simulink model "gm_Delay_compensation_FCS_MPC_6Phase_PMSM"  (R2022a)
settings: Solver=FixedStepDiscrete  StartTime=0.0  StopTime=10.0  RelTol=1e-3
undefined symbols (not defined in the file or in its folder): f_c, L_d, L_q, L_x, L_y, p, psi_pm, R_ph
libraries: hdlmdlgenlib x5
settings Model: Creator=Andre Merx  LastModifiedBy=Andre Merx
settings SolverCC: AlgebraicLoopSolver=TrustRegion
settings DataIOCC: LimitDataPoints=on  SaveOutput=off  SaveTime=off
settings OptimizationCC: BlockReduction=off  ConditionallyExecuteInputs=off  DefaultParameterBehavior=Inlined  LifeSpan=inf
settings DebuggingCC: AlgebraicLoopMsg=error  InheritedTsInSrcMsg=none  SingleTaskRateTransMsg=error  UnconnectedInputMsg=warning  UnconnectedOutputMsg=warning  UnconnectedLineMsg=warning  AllowSymbolicDim=off  StrictBusMsg=ErrorOnBusTreatedAsVector  SFUnexpectedBacktrackingDiag=warning  SFNoUnconditionalDefaultTransitionDiag=warning  SFExecutionAtInitializationDiag=none  SFMachineParentedDataDiag=warning  ArithmeticOperatorsInVariantConditions=warning
settings HardwareCC: ProdBitPerPointer=32  ProdBitPerSizeT=32  ProdBitPerPtrDiffT=32  ProdLargestAtomicFloat=None  ProdIntDivRoundTo=Undefined  ProdEndianess=Unspecified  ProdWordSize=32  ProdHWDeviceType=ASIC/FPGA->ASIC/FPGA  ProdEqTarget=off
settings SFSimCC: SimUseLocalCustomCode=off  CustomCodeUndefinedFunction=UseInterfaceOnly
settings RTWCC: RTWUseLocalCustomCode=off
settings CodeAppCC: StateflowObjectComments=on
settings GRTTargetCC: TargetLangStandard=C89/C90 (ANSI)
settings ConfigComp: CovScope=ReferencedModels  CovMetricSettings=dw  CovSaveCumulativeToWorkspaceVar=on  CovSaveSingleToWorkspaceVar=on  CovExternalEMLEnable=off  CovSFcnEnable=off

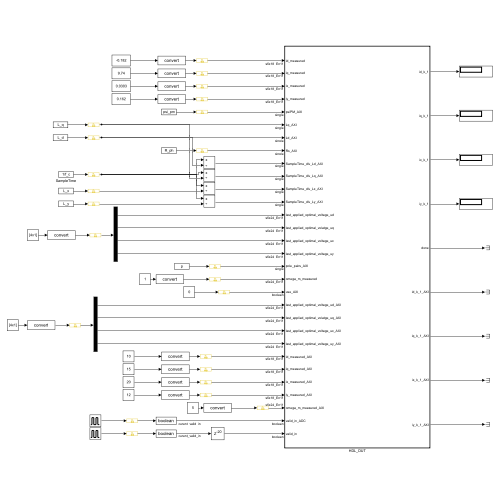
[thumbnail: Simulink's stored preview of the top-level diagram]
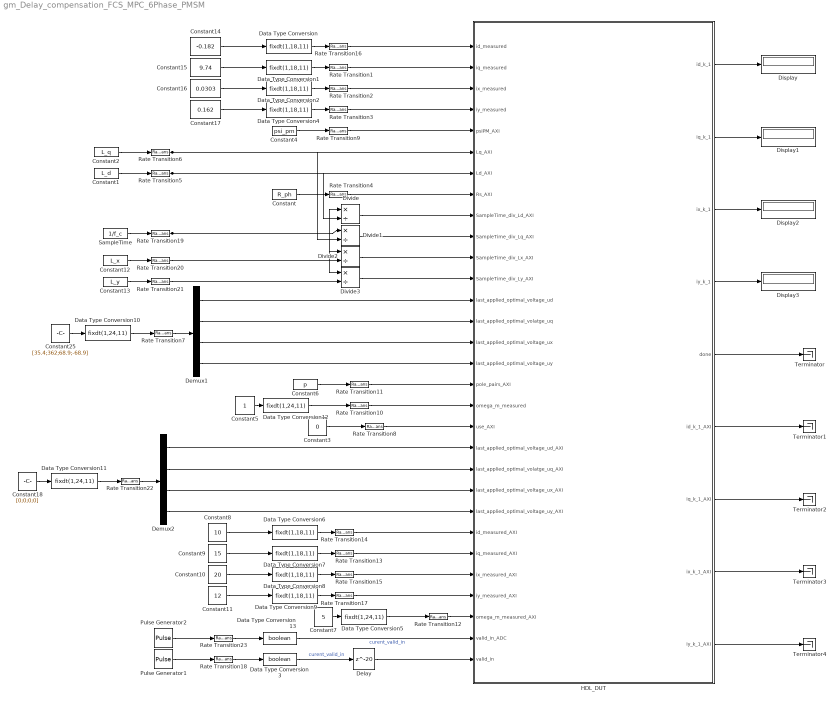
== system gm_Delay_compensation_FCS_MPC_6Phase_PMSM ==
  Constant : Constant  Value=R_ph  OutDataTypeStr=single  SampleTime=-1
  Constant1 : Constant  Value=L_d  OutDataTypeStr=single  SampleTime=-1
  Constant10 : Constant  Value=20
  Constant11 : Constant  Value=12
  Constant12 : Constant  Value=L_x  OutDataTypeStr=single  SampleTime=-1
  Constant13 : Constant  Value=L_y  OutDataTypeStr=single  SampleTime=-1
  Constant14 : Constant  Value=-0.182
  Constant15 : Constant  Value=9.74
  Constant16 : Constant  Value=0.0303
  Constant17 : Constant  Value=0.162
  Constant18 : Constant  Value=[0;0;0;0]
  Constant2 : Constant  Value=L_q  OutDataTypeStr=single  SampleTime=-1
  Constant25 : Constant  Value=[35.4;362;68.9;-68.9]
  Constant3 : Constant  Value=0  OutDataTypeStr=boolean  SampleTime=-1
  Constant4 : Constant  Value=psi_pm  OutDataTypeStr=single  SampleTime=-1
  Constant5 : Constant
  Constant6 : Constant  Value=p  OutDataTypeStr=single  SampleTime=-1
  Constant7 : Constant  Value=5
  Constant8 : Constant  Value=10
  Constant9 : Constant  Value=15
  Data Type Conversion{,1..2,4,6..9} (8 alike) : DataTypeConversion  OutDataTypeStr=fixdt(1,18,11)  SaturateOnIntegerOverflow=off  RndMeth=Floor
  Data Type Conversion{5,10..12} (4 alike) : DataTypeConversion  OutDataTypeStr=fixdt(1,24,11)  SaturateOnIntegerOverflow=off  RndMeth=Floor
  Data Type Conversion13 : DataTypeConversion  OutDataTypeStr=boolean  SaturateOnIntegerOverflow=off  RndMeth=Floor
  Data Type Conversion3 : DataTypeConversion  OutDataTypeStr=boolean  SaturateOnIntegerOverflow=off  RndMeth=Floor
  Delay : Delay  DelayLength=20
  Demux1 : Demux
  Demux2 : Demux
  Display{,1..3} (4 alike) : Display
  Divide{,1..3} (4 alike) : Product  Inputs=*/  RndMeth=Zero  SaturateOnIntegerOverflow=on
  HDL_DUT : Subsystem  TreatAsAtomicUnit=on
  Pulse Generator1 : DiscretePulseGenerator  PulseType=Time based  Period=1/f_c
  Pulse Generator2 : DiscretePulseGenerator  PulseType=Time based  Period=1/f_c
  Rate Transition{1..23} (23 alike) : RateTransition  OutPortSampleTime=Rt
  SampleTime : Constant  Value=1/f_c  OutDataTypeStr=single  SampleTime=-1
  Terminator{,1..4} (5 alike) : Terminator
  wires:
  Delay/1 -> HDL_DUT/30(valid_in)
  Data Type Conversion13/1 -> HDL_DUT/29(valid_in_ADC)  "curent_valid_in"
  Rate Transition23/1 -> Data Type Conversion13/1
  Pulse Generator2/1 -> Rate Transition23/1
  HDL_DUT/9(iy_k_1_AXI) -> Terminator4/1
  HDL_DUT/8(ix_k_1_AXI) -> Terminator3/1
  HDL_DUT/7(iq_k_1_AXI) -> Terminator2/1
  HDL_DUT/6(id_k_1_AXI) -> Terminator1/1
  Data Type Conversion11/1 -> Rate Transition22/1
  Data Type Conversion10/1 -> Rate Transition7/1
  Demux2/2 -> HDL_DUT/21(last_applied_optimal_volatge_uq_AXI)
  Demux2/4 -> HDL_DUT/23(last_applied_optimal_voltage_uy_AXI)
  Demux2/3 -> HDL_DUT/22(last_applied_optimal_voltage_ux_AXI)
  Demux2/1 -> HDL_DUT/20(last_applied_optimal_voltage_ud_AXI)
  Constant18/1 -> Data Type Conversion11/1
  Rate Transition22/1 -> Demux2/1
  Data Type Conversion7/1 -> Rate Transition13/1
  Constant9/1 -> Data Type Conversion7/1
  Rate Transition13/1 -> HDL_DUT/25(iq_measured_AXI)
  Rate Transition14/1 -> HDL_DUT/24(id_measured_AXI)
  Constant11/1 -> Data Type Conversion9/1
  Rate Transition17/1 -> HDL_DUT/27(iy_measured_AXI)
  Rate Transition15/1 -> HDL_DUT/26(ix_measured_AXI)
  Data Type Conversion9/1 -> Rate Transition17/1
  Constant8/1 -> Data Type Conversion6/1
  Data Type Conversion8/1 -> Rate Transition15/1
  Data Type Conversion6/1 -> Rate Transition14/1
  Constant10/1 -> Data Type Conversion8/1
  Rate Transition12/1 -> HDL_DUT/28(omega_m_measured_AXI)
  Data Type Conversion5/1 -> Rate Transition12/1
  Constant7/1 -> Data Type Conversion5/1
  Rate Transition8/1 -> HDL_DUT/19(use_AXI)
  Constant3/1 -> Rate Transition8/1
  HDL_DUT/5(done) -> Terminator/1
  HDL_DUT/4(iy_k_1) -> Display3/1
  HDL_DUT/3(ix_k_1) -> Display2/1
  HDL_DUT/2(iq_k_1) -> Display1/1
  HDL_DUT/1(id_k_1) -> Display/1
  Rate Transition7/1 -> Demux1/1
  Constant17/1 -> Data Type Conversion4/1
  Rate Transition16/1 -> HDL_DUT/1(id_measured)
  Constant15/1 -> Data Type Conversion1/1
  Rate Transition1/1 -> HDL_DUT/2(iq_measured)
  Data Type Conversion4/1 -> Rate Transition3/1
  Rate Transition4/1 -> HDL_DUT/8(Rs_AXI)
  Rate Transition5/1 -> HDL_DUT/7(Ld_AXI), Divide/2
  Constant6/1 -> Rate Transition11/1
  Demux1/4 -> HDL_DUT/16(last_applied_optimal_voltage_uy)
  Demux1/3 -> HDL_DUT/15(last_applied_optimal_voltage_ux)
  Constant16/1 -> Data Type Conversion2/1
  Data Type Conversion/1 -> Rate Transition16/1
  Constant4/1 -> Rate Transition9/1
  Data Type Conversion2/1 -> Rate Transition2/1
  Data Type Conversion1/1 -> Rate Transition1/1
  Constant14/1 -> Data Type Conversion/1
  Rate Transition3/1 -> HDL_DUT/4(iy_measured)
  Rate Transition2/1 -> HDL_DUT/3(ix_measured)
  Rate Transition10/1 -> HDL_DUT/18(omega_m_measured)
  Rate Transition9/1 -> HDL_DUT/5(psiPM_AXI)
  Constant5/1 -> Data Type Conversion12/1
  Data Type Conversion12/1 -> Rate Transition10/1
  Constant/1 -> Rate Transition4/1
  Rate Transition6/1 -> HDL_DUT/6(Lq_AXI), Divide1/2
  Constant1/1 -> Rate Transition5/1
  Constant2/1 -> Rate Transition6/1
  Data Type Conversion3/1 -> Delay/1  "curent_valid_in"
  Pulse Generator1/1 -> Rate Transition18/1
  Constant12/1 -> Rate Transition20/1
  Constant13/1 -> Rate Transition21/1
  Rate Transition19/1 -> Divide/1, Divide1/1, Divide2/1, Divide3/1
  Divide1/1 -> HDL_DUT/10(SampleTime_div_Lq_AXI)
  Rate Transition11/1 -> HDL_DUT/17(pole_pairs_AXI)
  Rate Transition20/1 -> Divide2/2
  Divide3/1 -> HDL_DUT/12(SampleTime_div_Ly_AXI)
  Rate Transition18/1 -> Data Type Conversion3/1
  Rate Transition21/1 -> Divide3/2
  Divide2/1 -> HDL_DUT/11(SampleTime_div_Lx_AXI)
  SampleTime/1 -> Rate Transition19/1
  Divide/1 -> HDL_DUT/9(SampleTime_div_Ld_AXI)
  Constant25/1 -> Data Type Conversion10/1
  Demux1/1 -> HDL_DUT/13(last_applied_optimal_voltage_ud)
  Demux1/2 -> HDL_DUT/14(last_applied_optimal_volatge_uq)

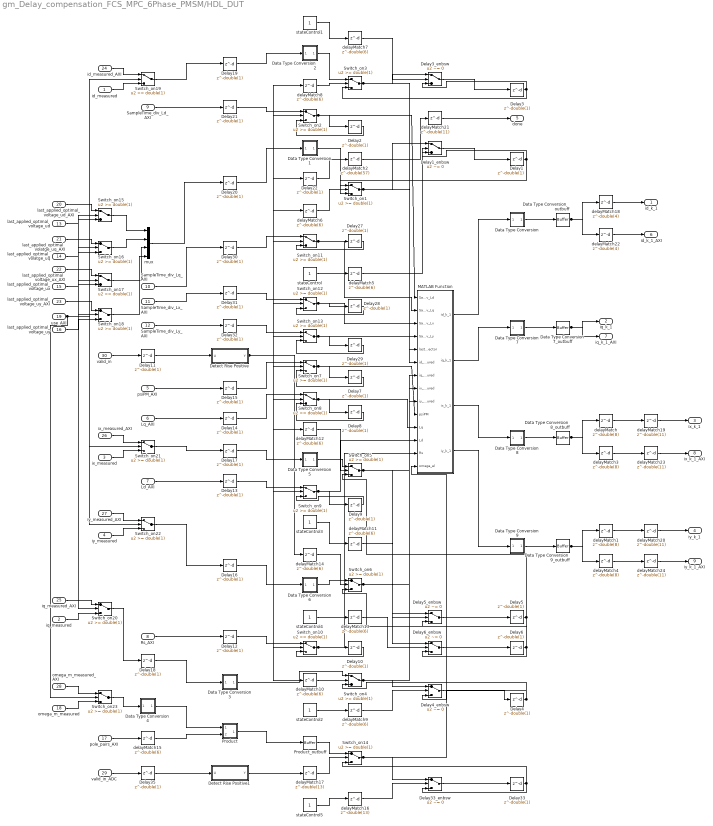
== system gm_Delay_compensation_FCS_MPC_6Phase_PMSM/HDL_DUT ==
  id_measured : Inport  OutDataTypeStr=fixdt(1, 18, 11)  PortDimensions=1  SampleTime=1e-08
  iq_measured : Inport  Port=2  OutDataTypeStr=fixdt(1, 18, 11)  PortDimensions=1  SampleTime=1e-08
  ix_measured : Inport  Port=3  OutDataTypeStr=fixdt(1, 18, 11)  PortDimensions=1  SampleTime=1e-08
  iy_measured : Inport  Port=4  OutDataTypeStr=fixdt(1, 18, 11)  PortDimensions=1  SampleTime=1e-08
  psiPM_AXI : Inport  Port=5  OutDataTypeStr=single  PortDimensions=1  SampleTime=1e-08
  Lq_AXI : Inport  Port=6  OutDataTypeStr=single  PortDimensions=1  SampleTime=1e-08
  Ld_AXI : Inport  Port=7  OutDataTypeStr=single  PortDimensions=1  SampleTime=1e-08
  Rs_AXI : Inport  Port=8  OutDataTypeStr=single  PortDimensions=1  SampleTime=1e-08
  SampleTime_div_Ld_AXI : Inport  Port=9  OutDataTypeStr=single  PortDimensions=1  SampleTime=1e-08
  SampleTime_div_Lq_AXI : Inport  Port=10  OutDataTypeStr=single  PortDimensions=1  SampleTime=1e-08
  SampleTime_div_Lx_AXI : Inport  Port=11  OutDataTypeStr=single  PortDimensions=1  SampleTime=1e-08
  SampleTime_div_Ly_AXI : Inport  Port=12  OutDataTypeStr=single  PortDimensions=1  SampleTime=1e-08
  last_applied_optimal_voltage_ud : Inport  Port=13  OutDataTypeStr=fixdt(1, 24, 11)  PortDimensions=1  SampleTime=1e-08
  last_applied_optimal_volatge_uq : Inport  Port=14  OutDataTypeStr=fixdt(1, 24, 11)  PortDimensions=1  SampleTime=1e-08
  last_applied_optimal_voltage_ux : Inport  Port=15  OutDataTypeStr=fixdt(1, 24, 11)  PortDimensions=1  SampleTime=1e-08
  last_applied_optimal_voltage_uy : Inport  Port=16  OutDataTypeStr=fixdt(1, 24, 11)  PortDimensions=1  SampleTime=1e-08
  pole_pairs_AXI : Inport  Port=17  OutDataTypeStr=single  PortDimensions=1  SampleTime=1e-08
  omega_m_measured : Inport  Port=18  OutDataTypeStr=fixdt(1, 24, 11)  PortDimensions=1  SampleTime=1e-08
  use_AXI : Inport  Port=19  OutDataTypeStr=boolean  PortDimensions=1  SampleTime=1e-08
  last_applied_optimal_voltage_ud_AXI : Inport  Port=20  OutDataTypeStr=fixdt(1, 24, 11)  PortDimensions=1  SampleTime=1e-08
  last_applied_optimal_volatge_uq_AXI : Inport  Port=21  OutDataTypeStr=fixdt(1, 24, 11)  PortDimensions=1  SampleTime=1e-08
  last_applied_optimal_voltage_ux_AXI : Inport  Port=22  OutDataTypeStr=fixdt(1, 24, 11)  PortDimensions=1  SampleTime=1e-08
  last_applied_optimal_voltage_uy_AXI : Inport  Port=23  OutDataTypeStr=fixdt(1, 24, 11)  PortDimensions=1  SampleTime=1e-08
  id_measured_AXI : Inport  Port=24  OutDataTypeStr=fixdt(1, 18, 11)  PortDimensions=1  SampleTime=1e-08
  iq_measured_AXI : Inport  Port=25  OutDataTypeStr=fixdt(1, 18, 11)  PortDimensions=1  SampleTime=1e-08
  ix_measured_AXI : Inport  Port=26  OutDataTypeStr=fixdt(1, 18, 11)  PortDimensions=1  SampleTime=1e-08
  iy_measured_AXI : Inport  Port=27  OutDataTypeStr=fixdt(1, 18, 11)  PortDimensions=1  SampleTime=1e-08
  omega_m_measured_AXI : Inport  Port=28  OutDataTypeStr=fixdt(1, 24, 11)  PortDimensions=1  SampleTime=1e-08
  valid_in_ADC : Inport  Port=29  OutDataTypeStr=boolean  PortDimensions=1  SampleTime=1e-08
  valid_in : Inport  Port=30  OutDataTypeStr=boolean  PortDimensions=1  SampleTime=1e-08
  Data Type Conversion : Subsystem
      mask Display: disp('NFP\nconv');
  Data Type Conversion1 : Subsystem
      mask Display: disp('NFP\nconv');
  Data Type Conversion2 : Subsystem
      mask Display: disp('NFP\nconv');
  Data Type Conversion3 : Subsystem
      mask Display: disp('NFP\nconv');
  Data Type Conversion4 : Subsystem
      mask Display: disp('NFP\nconv');
  Data Type Conversion5 : Subsystem
      mask Display: disp('NFP\nconv');
  Data Type Conversion6 : Subsystem
      mask Display: disp('NFP\nconv');
  Data Type Conversion7 : Subsystem
      mask Display: disp('NFP\nconv');
  Data Type Conversion7_outbuff : hdlmdlgenlib/Buffer
      settings: SourceProductBaseCode=SL
  Data Type Conversion8 : Subsystem
      mask Display: disp('NFP\nconv');
  Data Type Conversion8_outbuff : hdlmdlgenlib/Buffer
      settings: SourceProductBaseCode=SL
  Data Type Conversion9 : Subsystem
      mask Display: disp('NFP\nconv');
  Data Type Conversion9_outbuff : hdlmdlgenlib/Buffer
      settings: SourceProductBaseCode=SL
  Data Type Conversion_outbuff : hdlmdlgenlib/Buffer
      settings: SourceProductBaseCode=SL
  Delay{1..22,27..33,35} (30 alike) : Delay  DelayLength=double(1)  InitialCondition=0  SampleTime=1e-08
  Delay1_enbsw : Switch  Criteria=u2 ~= 0  Threshold=double(0)  OutDataTypeStr=single  SampleTime=1e-08  SaturateOnIntegerOverflow=off  InputSameDT=off
  Delay33_enbsw : Switch  Criteria=u2 ~= 0  Threshold=double(0)  OutDataTypeStr=single  SampleTime=1e-08  SaturateOnIntegerOverflow=off  InputSameDT=off
  Delay3_enbsw : Switch  Criteria=u2 ~= 0  Threshold=double(0)  OutDataTypeStr=single  SampleTime=1e-08  SaturateOnIntegerOverflow=off  InputSameDT=off
  Delay4_enbsw : Switch  Criteria=u2 ~= 0  Threshold=double(0)  OutDataTypeStr=single  SampleTime=1e-08  SaturateOnIntegerOverflow=off  InputSameDT=off
  Delay5_enbsw : Switch  Criteria=u2 ~= 0  Threshold=double(0)  OutDataTypeStr=single  SampleTime=1e-08  SaturateOnIntegerOverflow=off  InputSameDT=off
  Delay6_enbsw : Switch  Criteria=u2 ~= 0  Threshold=double(0)  OutDataTypeStr=single  SampleTime=1e-08  SaturateOnIntegerOverflow=off  InputSameDT=off
  Detect Rise Positive : Subsystem  mask(Detect Rise Positive){vinit=double(0), InputProcessing=Elements as channels (sample based), OutDataTypeStr=boolean}
      mask prompts: vinit "Simulink:masks:InitialCondition_MP"; InputProcessing "Simulink:masks:InputProcessing_MP"; OutDataTypeStr "Simulink:masks:OutputDataType_MP"
      mask help: Simulink:masks:DetectRisePositive_MD
      mask init:
      | InputProcessing = 'Elements as channels (sample based)';
      | OutDataTypeStr = 'boolean';
      | vinit = double(0);
      mask TypeOptions InputProcessing: Simulink:masks:ColumnsAsChannelsFrameBased | Simulink:masks:ElementsAsChannelsSampleBased
      mask TypeOptions OutDataTypeStr: Simulink:masks:uint8 | Simulink:masks:boolean
      mask Display: fprintf('U > 0\n&  NOT\nU/z > 0')
  Detect Rise Positive1 : Subsystem  mask(Detect Rise Positive){vinit=double(0), InputProcessing=Elements as channels (sample based), OutDataTypeStr=boolean}
      mask prompts: vinit "Simulink:masks:InitialCondition_MP"; InputProcessing "Simulink:masks:InputProcessing_MP"; OutDataTypeStr "Simulink:masks:OutputDataType_MP"
      mask help: Simulink:masks:DetectRisePositive_MD
      mask init:
      | InputProcessing = 'Elements as channels (sample based)';
      | OutDataTypeStr = 'boolean';
      | vinit = double(0);
      mask TypeOptions InputProcessing: Simulink:masks:ColumnsAsChannelsFrameBased | Simulink:masks:ElementsAsChannelsSampleBased
      mask TypeOptions OutDataTypeStr: Simulink:masks:uint8 | Simulink:masks:boolean
      mask Display: fprintf('U > 0\n&  NOT\nU/z > 0')
  MATLAB Function : Subsystem
  Product : Subsystem
      mask Display: disp('NFP\nmul');
  Product_outbuff : hdlmdlgenlib/Buffer
      settings: SourceProductBaseCode=SL
  Switch_on{1..14} (14 alike) : Switch  Threshold=double(1)  OutDataTypeStr=single  RndMeth=Simplest  SampleTime=1e-08  SaturateOnIntegerOverflow=off  InputSameDT=off
  Switch_on{15..18,23} (5 alike) : Switch  Threshold=double(1)  OutDataTypeStr=fixdt(1, 24, 11)  RndMeth=Simplest  SampleTime=1e-08  SaturateOnIntegerOverflow=off  InputSameDT=off
  Switch_on{19..22} (4 alike) : Switch  Threshold=double(1)  OutDataTypeStr=fixdt(1, 18, 11)  RndMeth=Simplest  SampleTime=1e-08  SaturateOnIntegerOverflow=off  InputSameDT=off
  delayMatch{,1,3..4} (4 alike) : Delay  DelayLength=double(8)  InitialCondition=0  SampleTime=1e-08
  delayMatch{5..15} (11 alike) : Delay  DelayLength=double(6)  InitialCondition=0  SampleTime=1e-08
  delayMatch16 : Delay  DelayLength=double(13)  InitialCondition=0  SampleTime=1e-08
  delayMatch17 : Delay  DelayLength=double(13)  InitialCondition=0  SampleTime=1e-08
  delayMatch18 : Delay  DelayLength=double(4)  InitialCondition=0  SampleTime=1e-08
  delayMatch{19..21,23..24} (5 alike) : Delay  DelayLength=double(11)  InitialCondition=0  SampleTime=1e-08
  delayMatch2 : Delay  DelayLength=double(57)  InitialCondition=0  SampleTime=1e-08
  delayMatch22 : Delay  DelayLength=double(4)  InitialCondition=0  SampleTime=1e-08
  mux : Mux
  stateControl{,1..5} (6 alike) : Constant  OutDataTypeStr=boolean  SampleTime=1e-08
  id_k_1 : Outport  SampleTime=1e-08
  iq_k_1 : Outport  Port=2  SampleTime=1e-08
  ix_k_1 : Outport  Port=3  SampleTime=1e-08
  iy_k_1 : Outport  Port=4  SampleTime=1e-08
  done : Outport  Port=5  SampleTime=1e-08
  id_k_1_AXI : Outport  Port=6  SampleTime=1e-08
  iq_k_1_AXI : Outport  Port=7  SampleTime=1e-08
  ix_k_1_AXI : Outport  Port=8  SampleTime=1e-08
  iy_k_1_AXI : Outport  Port=9  SampleTime=1e-08
  wires:
  id_measured/1 -> Switch_on19/3
  iq_measured/1 -> Switch_on20/3
  ix_measured/1 -> Switch_on21/3
  iy_measured/1 -> Switch_on22/3
  psiPM_AXI/1 -> Delay15/1
  Lq_AXI/1 -> Delay14/1
  Ld_AXI/1 -> Delay13/1
  Rs_AXI/1 -> Delay12/1
  SampleTime_div_Ld_AXI/1 -> Delay21/1
  SampleTime_div_Lq_AXI/1 -> Delay30/1
  SampleTime_div_Lx_AXI/1 -> Delay31/1
  SampleTime_div_Ly_AXI/1 -> Delay32/1
  last_applied_optimal_voltage_ud/1 -> Switch_on15/3
  last_applied_optimal_volatge_uq/1 -> Switch_on16/3
  last_applied_optimal_voltage_ux/1 -> Switch_on17/3
  last_applied_optimal_voltage_uy/1 -> Switch_on18/3
  delayMatch15/1 -> Product/2(In2)
  omega_m_measured/1 -> Switch_on23/3
  use_AXI/1 -> Switch_on23/2, Switch_on22/2, Switch_on21/2, Switch_on20/2, Switch_on19/2, Switch_on18/2, Switch_on17/2, Switch_on16/2, Switch_on15/2
  last_applied_optimal_voltage_ud_AXI/1 -> Switch_on15/1
  last_applied_optimal_volatge_uq_AXI/1 -> Switch_on16/1
  last_applied_optimal_voltage_ux_AXI/1 -> Switch_on17/1
  last_applied_optimal_voltage_uy_AXI/1 -> Switch_on18/1
  id_measured_AXI/1 -> Switch_on19/1
  iq_measured_AXI/1 -> Switch_on20/1
  ix_measured_AXI/1 -> Switch_on21/1
  iy_measured_AXI/1 -> Switch_on22/1
  omega_m_measured_AXI/1 -> Switch_on23/1
  valid_in_ADC/1 -> Delay35/1
  valid_in/1 -> Delay11/1
  Data Type Conversion_outbuff/1 -> delayMatch18/1, delayMatch22/1
  Data Type Conversion7_outbuff/1 -> iq_k_1_AXI/1, iq_k_1/1
  Data Type Conversion8_outbuff/1 -> delayMatch3/1, delayMatch/1
  Data Type Conversion9_outbuff/1 -> delayMatch4/1, delayMatch1/1
  Delay11/1 -> Detect Rise Positive/1(U)
  Delay12/1 -> Switch_on10/1
  Delay13/1 -> Switch_on9/1
  Delay14/1 -> Switch_on8/1
  Delay15/1 -> Switch_on7/1
  Delay16/1 -> Data Type Conversion6/1(In1)
  Delay17/1 -> Data Type Conversion5/1(In1)
  Delay18/1 -> Data Type Conversion3/1(In1)
  Delay19/1 -> Data Type Conversion2/1(In1)
  Delay20/1 -> Data Type Conversion1/1(In1)
  Delay21/1 -> Switch_on2/1
  delayMatch21/1 -> done/1
  delayMatch20/1 -> iy_k_1/1
  delayMatch19/1 -> ix_k_1/1
  delayMatch18/1 -> id_k_1/1
  Delay30/1 -> Switch_on11/1
  Delay31/1 -> Switch_on12/1
  Delay32/1 -> Switch_on13/1
  Delay35/1 -> Detect Rise Positive1/1(U)
  delayMatch6/1 -> Switch_on1/2
  delayMatch17/1 -> Switch_on14/2
  MATLAB Function/1(id_k_1) -> Data Type Conversion/1(In1)
  MATLAB Function/2(iq_k_1) -> Data Type Conversion7/1(In1)
  MATLAB Function/3(ix_k_1) -> Data Type Conversion8/1(In1)
  MATLAB Function/4(iy_k_1) -> Data Type Conversion9/1(In1)
  mux/1 -> Delay20/1
  Product_outbuff/1 -> Switch_on14/1
  Switch_on10/1 -> MATLAB Function/13(Rs), Delay10/1
  Switch_on11/1 -> MATLAB Function/2(SampleTime_div_Lq), Delay27/1
  Switch_on12/1 -> MATLAB Function/3(SampleTime_div_Lx), Delay28/1
  Switch_on13/1 -> MATLAB Function/4(SampleTime_div_Ly), Delay29/1
  Switch_on15/1 -> mux/1
  Switch_on16/1 -> mux/2
  Switch_on17/1 -> mux/3
  Switch_on18/1 -> mux/4
  Switch_on19/1 -> Delay19/1
  Switch_on2/1 -> MATLAB Function/1(SampleTime_div_Ld), Delay2/1
  Switch_on20/1 -> Delay18/1
  Switch_on21/1 -> Delay17/1
  Switch_on22/1 -> Delay16/1
  Switch_on23/1 -> Data Type Conversion4/1(In1)
  Switch_on7/1 -> MATLAB Function/10(psiPM), Delay7/1
  Switch_on8/1 -> MATLAB Function/11(Lq), Delay8/1
  Switch_on9/1 -> MATLAB Function/12(Ld), Delay9/1
  delayMatch22/1 -> id_k_1_AXI/1
  delayMatch23/1 -> ix_k_1_AXI/1
  delayMatch24/1 -> iy_k_1_AXI/1
  Delay22/1 -> delayMatch2/1
  Data Type Conversion/1(Out1) -> Data Type Conversion_outbuff/1
  Data Type Conversion1/1(Out1) -> Switch_on1/1
  Data Type Conversion2/1(Out1) -> Switch_on3/1
  Data Type Conversion3/1(Out1) -> Switch_on4/1
  Data Type Conversion4/1(Out1) -> Product/1(In1)
  Data Type Conversion5/1(Out1) -> Switch_on5/1
  Data Type Conversion6/1(Out1) -> Switch_on6/1
  Data Type Conversion7/1(Out1) -> Data Type Conversion7_outbuff/1
  Data Type Conversion8/1(Out1) -> Data Type Conversion8_outbuff/1
  Data Type Conversion9/1(Out1) -> Data Type Conversion9_outbuff/1
  Product/1(Out1) -> Product_outbuff/1
  delayMatch5/1 -> Delay1_enbsw/2
  delayMatch7/1 -> Delay3_enbsw/2
  delayMatch9/1 -> Delay4_enbsw/2
  delayMatch11/1 -> Delay5_enbsw/2
  delayMatch13/1 -> Delay6_enbsw/2
  delayMatch16/1 -> Delay33_enbsw/2
  stateControl/1 -> delayMatch5/1
  delayMatch8/1 -> Switch_on3/2
  stateControl1/1 -> delayMatch7/1
  delayMatch10/1 -> Switch_on4/2
  stateControl2/1 -> delayMatch9/1
  delayMatch12/1 -> Switch_on5/2
  stateControl3/1 -> delayMatch11/1
  delayMatch14/1 -> Switch_on6/2
  stateControl4/1 -> delayMatch13/1
  Detect Rise Positive/1(Y) -> delayMatch14/1, delayMatch12/1, delayMatch10/1, delayMatch8/1, delayMatch6/1, Delay22/1, Switch_on2/2, Switch_on11/2, Switch_on12/2, Switch_on13/2, Switch_on7/2, Switch_on8/2, Switch_on9/2, Switch_on10/2
  pole_pairs_AXI/1 -> delayMatch15/1
  stateControl5/1 -> delayMatch16/1
  Detect Rise Positive1/1(Y) -> delayMatch17/1
  delayMatch/1 -> delayMatch19/1
  delayMatch1/1 -> delayMatch20/1
  delayMatch2/1 -> delayMatch21/1
  delayMatch3/1 -> delayMatch23/1
  delayMatch4/1 -> delayMatch24/1
  Switch_on1/1 -> MATLAB Function/5(last_applied_optimal_voltage_vector), Delay1_enbsw/1
  Switch_on3/1 -> MATLAB Function/6(id_measured), Delay3_enbsw/1
  Switch_on4/1 -> MATLAB Function/7(iq_measured), Delay4_enbsw/1
  Switch_on5/1 -> MATLAB Function/8(ix_measured), Delay5_enbsw/1
  Switch_on6/1 -> MATLAB Function/9(iy_measured), Delay6_enbsw/1
  Switch_on14/1 -> MATLAB Function/14(omega_el), Delay33_enbsw/1
  Delay2/1 -> Switch_on2/3
  Delay27/1 -> Switch_on11/3
  Delay28/1 -> Switch_on12/3
  Delay29/1 -> Switch_on13/3
  Delay1_enbsw/1 -> Delay1/1
  Delay1/1 -> Switch_on1/3, Delay1_enbsw/3
  Delay3_enbsw/1 -> Delay3/1
  Delay3/1 -> Switch_on3/3, Delay3_enbsw/3
  Delay4_enbsw/1 -> Delay4/1
  Delay4/1 -> Switch_on4/3, Delay4_enbsw/3
  Delay5_enbsw/1 -> Delay5/1
  Delay5/1 -> Switch_on5/3, Delay5_enbsw/3
  Delay6_enbsw/1 -> Delay6/1
  Delay6/1 -> Switch_on6/3, Delay6_enbsw/3
  Delay7/1 -> Switch_on7/3
  Delay8/1 -> Switch_on8/3
  Delay9/1 -> Switch_on9/3
  Delay10/1 -> Switch_on10/3
  Delay33_enbsw/1 -> Delay33/1
  Delay33/1 -> Switch_on14/3, Delay33_enbsw/3

== system gm_Delay_compensation_FCS_MPC_6Phase_PMSM/HDL_DUT/Data Type Conversion ==
  In1 : Inport
  Data Type Conversion : DataTypeConversion  OutDataTypeStr=fixdt(1, 18, 11)  SampleTime=1e-08  SaturateOnIntegerOverflow=off  RndMeth=Floor
  Data Type Conversion_pd1 : Delay  DelayLength=6
  Out1 : Outport
  wires:
  In1/1 -> Data Type Conversion/1
  Data Type Conversion/1 -> Data Type Conversion_pd1/1
  Data Type Conversion_pd1/1 -> Out1/1

== system gm_Delay_compensation_FCS_MPC_6Phase_PMSM/HDL_DUT/Data Type Conversion1 ==
  In1 : Inport
  Data Type Conversion1 : DataTypeConversion  OutDataTypeStr=single  RndMeth=Nearest  SampleTime=1e-08  SaturateOnIntegerOverflow=off
  Data Type Conversion1_pd1 : Delay  DelayLength=6
  Out1 : Outport
  wires:
  In1/1 -> Data Type Conversion1/1
  Data Type Conversion1/1 -> Data Type Conversion1_pd1/1
  Data Type Conversion1_pd1/1 -> Out1/1

== system gm_Delay_compensation_FCS_MPC_6Phase_PMSM/HDL_DUT/Data Type Conversion2 ==
  In1 : Inport
  Data Type Conversion2 : DataTypeConversion  OutDataTypeStr=single  RndMeth=Nearest  SampleTime=1e-08  SaturateOnIntegerOverflow=off
  Data Type Conversion2_pd1 : Delay  DelayLength=6
  Out1 : Outport
  wires:
  In1/1 -> Data Type Conversion2/1
  Data Type Conversion2/1 -> Data Type Conversion2_pd1/1
  Data Type Conversion2_pd1/1 -> Out1/1

== system gm_Delay_compensation_FCS_MPC_6Phase_PMSM/HDL_DUT/Data Type Conversion3 ==
  In1 : Inport
  Data Type Conversion3 : DataTypeConversion  OutDataTypeStr=single  RndMeth=Nearest  SampleTime=1e-08  SaturateOnIntegerOverflow=off
  Data Type Conversion3_pd1 : Delay  DelayLength=6
  Out1 : Outport
  wires:
  In1/1 -> Data Type Conversion3/1
  Data Type Conversion3/1 -> Data Type Conversion3_pd1/1
  Data Type Conversion3_pd1/1 -> Out1/1

== system gm_Delay_compensation_FCS_MPC_6Phase_PMSM/HDL_DUT/Data Type Conversion4 ==
  In1 : Inport
  Data Type Conversion4 : DataTypeConversion  OutDataTypeStr=single  RndMeth=Nearest  SampleTime=1e-08  SaturateOnIntegerOverflow=off
  Data Type Conversion4_pd1 : Delay  DelayLength=6
  Out1 : Outport
  wires:
  In1/1 -> Data Type Conversion4/1
  Data Type Conversion4/1 -> Data Type Conversion4_pd1/1
  Data Type Conversion4_pd1/1 -> Out1/1

== system gm_Delay_compensation_FCS_MPC_6Phase_PMSM/HDL_DUT/Data Type Conversion5 ==
  In1 : Inport
  Data Type Conversion5 : DataTypeConversion  OutDataTypeStr=single  RndMeth=Nearest  SampleTime=1e-08  SaturateOnIntegerOverflow=off
  Data Type Conversion5_pd1 : Delay  DelayLength=6
  Out1 : Outport
  wires:
  In1/1 -> Data Type Conversion5/1
  Data Type Conversion5/1 -> Data Type Conversion5_pd1/1
  Data Type Conversion5_pd1/1 -> Out1/1

== system gm_Delay_compensation_FCS_MPC_6Phase_PMSM/HDL_DUT/Data Type Conversion6 ==
  In1 : Inport
  Data Type Conversion6 : DataTypeConversion  OutDataTypeStr=single  RndMeth=Nearest  SampleTime=1e-08  SaturateOnIntegerOverflow=off
  Data Type Conversion6_pd1 : Delay  DelayLength=6
  Out1 : Outport
  wires:
  In1/1 -> Data Type Conversion6/1
  Data Type Conversion6/1 -> Data Type Conversion6_pd1/1
  Data Type Conversion6_pd1/1 -> Out1/1

== system gm_Delay_compensation_FCS_MPC_6Phase_PMSM/HDL_DUT/Data Type Conversion7 ==
  In1 : Inport
  Data Type Conversion7 : DataTypeConversion  OutDataTypeStr=fixdt(1, 18, 11)  SampleTime=1e-08  SaturateOnIntegerOverflow=off  RndMeth=Floor
  Data Type Conversion7_pd1 : Delay  DelayLength=6
  Out1 : Outport
  wires:
  In1/1 -> Data Type Conversion7/1
  Data Type Conversion7/1 -> Data Type Conversion7_pd1/1
  Data Type Conversion7_pd1/1 -> Out1/1

== system gm_Delay_compensation_FCS_MPC_6Phase_PMSM/HDL_DUT/Data Type Conversion8 ==
  In1 : Inport
  Data Type Conversion8 : DataTypeConversion  OutDataTypeStr=fixdt(1, 18, 11)  SampleTime=1e-08  SaturateOnIntegerOverflow=off  RndMeth=Floor
  Data Type Conversion8_pd1 : Delay  DelayLength=6
  Out1 : Outport
  wires:
  In1/1 -> Data Type Conversion8/1
  Data Type Conversion8/1 -> Data Type Conversion8_pd1/1
  Data Type Conversion8_pd1/1 -> Out1/1

== system gm_Delay_compensation_FCS_MPC_6Phase_PMSM/HDL_DUT/Data Type Conversion9 ==
  In1 : Inport
  Data Type Conversion9 : DataTypeConversion  OutDataTypeStr=fixdt(1, 18, 11)  SampleTime=1e-08  SaturateOnIntegerOverflow=off  RndMeth=Floor
  Data Type Conversion9_pd1 : Delay  DelayLength=6
  Out1 : Outport
  wires:
  In1/1 -> Data Type Conversion9/1
  Data Type Conversion9/1 -> Data Type Conversion9_pd1/1
  Data Type Conversion9_pd1/1 -> Out1/1

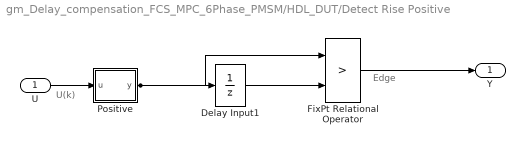
== system gm_Delay_compensation_FCS_MPC_6Phase_PMSM/HDL_DUT/Detect Rise Positive ==
  note: Edge
  note: U(k)
  U : Inport  OutDataTypeStr=boolean  SampleTime=1e-08
  Delay Input1 : UnitDelay  Description=Store in Global RAM  DisableCoverage=on  InitialCondition=vinit  SampleTime=-1  HasFrameUpgradeWarning=on
  FixPt Relational Operator : RelationalOperator  Operator=>  OutDataTypeStr=boolean  ZeroCross=off  InputSameDT=off
  Positive : Subsystem  mask(Compare To Zero){relop=>, OutDataTypeStr=boolean, ZeroCross=off}
      mask prompts: relop "Simulink:masks:Operator_MP"; OutDataTypeStr "Simulink:masks:OutputDataType_MP"; ZeroCross "Simulink:masks:EnableZerocrossingDetection_MP"
      mask help: Simulink:masks:CompareToZero_MD
      mask init:
      | OutDataTypeStr = 'boolean';
      | ZeroCross = 'off';
      | blkName = 'Delay_compensation_FCS_MPC_6Phase_PMSM/HDL_DUT/Detect Rise\nPositive/Positive';
      | relop = '>';
      | setValue = 'boolean';
      mask TypeOptions relop: == | ~= | < | <= | >= | >
      mask TypeOptions OutDataTypeStr: Simulink:masks:uint8 | Simulink:masks:boolean
      mask Callback ZeroCross: sl('zeroCrossEnable', gcbh);
      mask Display: disp([relop,' 0'])
  Y : Outport  SampleTime=1e-08
  wires:
  Delay Input1/1 -> FixPt Relational Operator/2
  FixPt Relational Operator/1 -> Y/1
  Positive/1(y) -> FixPt Relational Operator/1, Delay Input1/1
  U/1 -> Positive/1(u)

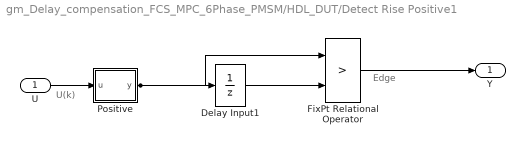
== system gm_Delay_compensation_FCS_MPC_6Phase_PMSM/HDL_DUT/Detect Rise Positive1 ==
  note: Edge
  note: U(k)
  U : Inport  OutDataTypeStr=boolean  SampleTime=1e-08
  Delay Input1 : UnitDelay  Description=Store in Global RAM  DisableCoverage=on  InitialCondition=vinit  SampleTime=-1  HasFrameUpgradeWarning=on
  FixPt Relational Operator : RelationalOperator  Operator=>  OutDataTypeStr=boolean  ZeroCross=off  InputSameDT=off
  Positive : Subsystem  mask(Compare To Zero){relop=>, OutDataTypeStr=boolean, ZeroCross=off}
      mask prompts: relop "Simulink:masks:Operator_MP"; OutDataTypeStr "Simulink:masks:OutputDataType_MP"; ZeroCross "Simulink:masks:EnableZerocrossingDetection_MP"
      mask help: Simulink:masks:CompareToZero_MD
      mask init:
      | OutDataTypeStr = 'boolean';
      | ZeroCross = 'off';
      | blkName = 'Delay_compensation_FCS_MPC_6Phase_PMSM/HDL_DUT/Detect Rise\nPositive1/Positive';
      | relop = '>';
      | setValue = 'boolean';
      mask TypeOptions relop: == | ~= | < | <= | >= | >
      mask TypeOptions OutDataTypeStr: Simulink:masks:uint8 | Simulink:masks:boolean
      mask Callback ZeroCross: sl('zeroCrossEnable', gcbh);
      mask Display: disp([relop,' 0'])
  Y : Outport  SampleTime=1e-08
  wires:
  Delay Input1/1 -> FixPt Relational Operator/2
  FixPt Relational Operator/1 -> Y/1
  Positive/1(y) -> FixPt Relational Operator/1, Delay Input1/1
  U/1 -> Positive/1(u)

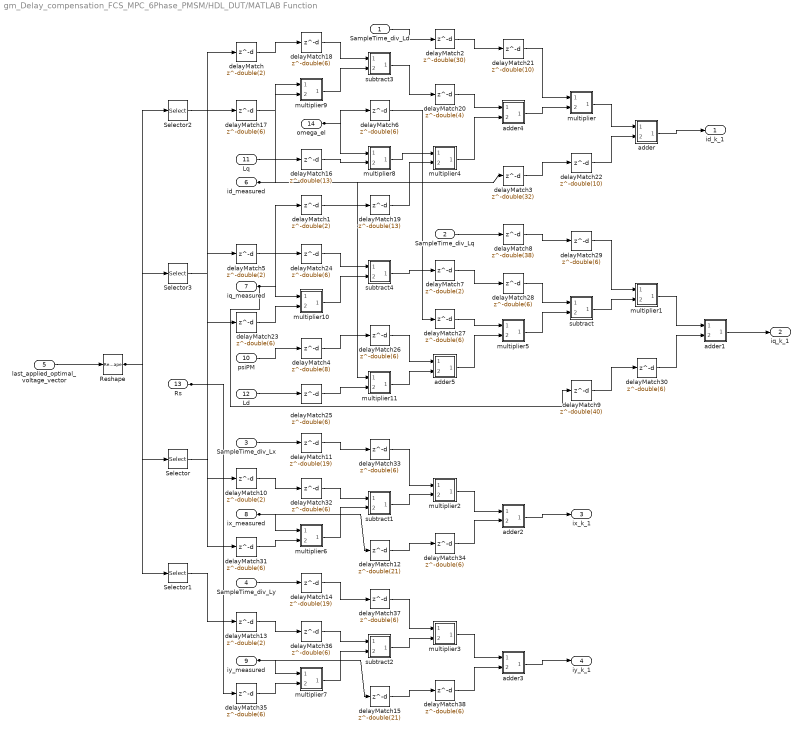
== system gm_Delay_compensation_FCS_MPC_6Phase_PMSM/HDL_DUT/MATLAB Function ==
  SampleTime_div_Ld : Inport  OutDataTypeStr=single  PortDimensions=1  SampleTime=1e-08
  SampleTime_div_Lq : Inport  Port=2  OutDataTypeStr=single  PortDimensions=1  SampleTime=1e-08
  SampleTime_div_Lx : Inport  Port=3  OutDataTypeStr=single  PortDimensions=1  SampleTime=1e-08
  SampleTime_div_Ly : Inport  Port=4  OutDataTypeStr=single  PortDimensions=1  SampleTime=1e-08
  last_applied_optimal_voltage_vector : Inport  Port=5  OutDataTypeStr=single  PortDimensions=[4]  SampleTime=1e-08
  id_measured : Inport  Port=6  OutDataTypeStr=single  PortDimensions=1  SampleTime=1e-08
  iq_measured : Inport  Port=7  OutDataTypeStr=single  PortDimensions=1  SampleTime=1e-08
  ix_measured : Inport  Port=8  OutDataTypeStr=single  PortDimensions=1  SampleTime=1e-08
  iy_measured : Inport  Port=9  OutDataTypeStr=single  PortDimensions=1  SampleTime=1e-08
  psiPM : Inport  Port=10  OutDataTypeStr=single  PortDimensions=1  SampleTime=1e-08
  Lq : Inport  Port=11  OutDataTypeStr=single  PortDimensions=1  SampleTime=1e-08
  Ld : Inport  Port=12  OutDataTypeStr=single  PortDimensions=1  SampleTime=1e-08
  Rs : Inport  Port=13  OutDataTypeStr=single  PortDimensions=1  SampleTime=1e-08
  omega_el : Inport  Port=14  OutDataTypeStr=single  PortDimensions=1  SampleTime=1e-08
  Reshape : Reshape  OutputDimensionality=Column vector (2-D)
  Selector : Selector  SampleTime=1e-08  IndexOptions=Index vector (dialog)  Indices=double(3)  OutputSizes=double(0)
  Selector1 : Selector  SampleTime=1e-08  IndexOptions=Index vector (dialog)  Indices=double(4)  OutputSizes=double(0)
  Selector2 : Selector  SampleTime=1e-08  IndexOptions=Index vector (dialog)  Indices=double(1)  OutputSizes=double(0)
  Selector3 : Selector  SampleTime=1e-08  IndexOptions=Index vector (dialog)  Indices=double(2)  OutputSizes=double(0)
  adder : Subsystem
      mask Display: disp('NFP\nadd');
  adder1 : Subsystem
      mask Display: disp('NFP\nadd');
  adder2 : Subsystem
      mask Display: disp('NFP\nadd');
  adder3 : Subsystem
      mask Display: disp('NFP\nadd');
  adder4 : Subsystem
      mask Display: disp('NFP\nadd');
  adder5 : Subsystem
      mask Display: disp('NFP\nadd');
  delayMatch{,1,5,7,10,13} (6 alike) : Delay  DelayLength=double(2)  InitialCondition=0  SampleTime=1e-08
  delayMatch11 : Delay  DelayLength=double(19)  InitialCondition=0  SampleTime=1e-08
  delayMatch12 : Delay  DelayLength=double(21)  InitialCondition=0  SampleTime=1e-08
  delayMatch14 : Delay  DelayLength=double(19)  InitialCondition=0  SampleTime=1e-08
  delayMatch15 : Delay  DelayLength=double(21)  InitialCondition=0  SampleTime=1e-08
  delayMatch16 : Delay  DelayLength=double(13)  InitialCondition=0  SampleTime=1e-08
  delayMatch{6,17..18,23..38} (19 alike) : Delay  DelayLength=double(6)  InitialCondition=0  SampleTime=1e-08
  delayMatch19 : Delay  DelayLength=double(13)  InitialCondition=0  SampleTime=1e-08
  delayMatch2 : Delay  DelayLength=double(30)  InitialCondition=0  SampleTime=1e-08
  delayMatch20 : Delay  DelayLength=double(4)  InitialCondition=0  SampleTime=1e-08
  delayMatch21 : Delay  DelayLength=double(10)  InitialCondition=0  SampleTime=1e-08
  delayMatch22 : Delay  DelayLength=double(10)  InitialCondition=0  SampleTime=1e-08
  delayMatch3 : Delay  DelayLength=double(32)  InitialCondition=0  SampleTime=1e-08
  delayMatch4 : Delay  DelayLength=double(8)  InitialCondition=0  SampleTime=1e-08
  delayMatch8 : Delay  DelayLength=double(38)  InitialCondition=0  SampleTime=1e-08
  delayMatch9 : Delay  DelayLength=double(40)  InitialCondition=0  SampleTime=1e-08
  multiplier : Subsystem
      mask Display: disp('NFP\nmul');
  multiplier1 : Subsystem
      mask Display: disp('NFP\nmul');
  multiplier10 : Subsystem
      mask Display: disp('NFP\nmul');
  multiplier11 : Subsystem
      mask Display: disp('NFP\nmul');
  multiplier2 : Subsystem
      mask Display: disp('NFP\nmul');
  multiplier3 : Subsystem
      mask Display: disp('NFP\nmul');
  multiplier4 : Subsystem
      mask Display: disp('NFP\nmul');
  multiplier5 : Subsystem
      mask Display: disp('NFP\nmul');
  multiplier6 : Subsystem
      mask Display: disp('NFP\nmul');
  multiplier7 : Subsystem
      mask Display: disp('NFP\nmul');
  multiplier8 : Subsystem
      mask Display: disp('NFP\nmul');
  multiplier9 : Subsystem
      mask Display: disp('NFP\nmul');
  subtract : Subsystem
      mask Display: disp('NFP\nadd');
  subtract1 : Subsystem
      mask Display: disp('NFP\nadd');
  subtract2 : Subsystem
      mask Display: disp('NFP\nadd');
  subtract3 : Subsystem
      mask Display: disp('NFP\nadd');
  subtract4 : Subsystem
      mask Display: disp('NFP\nadd');
  id_k_1 : Outport  SampleTime=1e-08  VectorParamsAs1DForOutWhenUnconnected=off
  iq_k_1 : Outport  Port=2  SampleTime=1e-08
  ix_k_1 : Outport  Port=3  SampleTime=1e-08
  iy_k_1 : Outport  Port=4  SampleTime=1e-08
  wires:
  delayMatch21/1 -> multiplier/1(In1)
  delayMatch29/1 -> multiplier1/1(In1)
  delayMatch33/1 -> multiplier2/1(In1)
  delayMatch37/1 -> multiplier3/1(In1)
  delayMatch22/1 -> adder/2(In2)
  delayMatch19/1 -> multiplier4/2(In2)
  delayMatch34/1 -> adder2/2(In2)
  delayMatch38/1 -> adder3/2(In2)
  delayMatch26/1 -> adder5/1(In1)
  delayMatch27/1 -> multiplier5/1(In1)
  delayMatch20/1 -> adder4/1(In1)
  delayMatch28/1 -> subtract/1(In1)
  delayMatch32/1 -> subtract1/1(In1)
  delayMatch36/1 -> subtract2/1(In1)
  delayMatch18/1 -> subtract3/1(In1)
  delayMatch24/1 -> subtract4/1(In1)
  Reshape/1 -> Selector3/1, Selector2/1, Selector1/1, Selector/1
  adder/1(Out1) -> id_k_1/1
  adder1/1(Out1) -> iq_k_1/1
  adder2/1(Out1) -> ix_k_1/1
  adder3/1(Out1) -> iy_k_1/1
  multiplier/1(Out1) -> adder/1(In1)
  multiplier1/1(Out1) -> adder1/1(In1)
  multiplier2/1(Out1) -> adder2/1(In1)
  multiplier3/1(Out1) -> adder3/1(In1)
  adder4/1(Out1) -> multiplier/2(In2)
  subtract/1(Out1) -> multiplier1/2(In2)
  subtract1/1(Out1) -> multiplier2/2(In2)
  subtract2/1(Out1) -> multiplier3/2(In2)
  multiplier4/1(Out1) -> adder4/2(In2)
  subtract3/1(Out1) -> delayMatch20/1
  multiplier5/1(Out1) -> subtract/2(In2)
  subtract4/1(Out1) -> delayMatch7/1
  multiplier6/1(Out1) -> subtract1/2(In2)
  multiplier7/1(Out1) -> subtract2/2(In2)
  multiplier8/1(Out1) -> multiplier4/1(In1)
  multiplier9/1(Out1) -> subtract3/2(In2)
  adder5/1(Out1) -> multiplier5/2(In2)
  multiplier10/1(Out1) -> subtract4/2(In2)
  multiplier11/1(Out1) -> adder5/2(In2)
  Selector2/1 -> delayMatch/1
  delayMatch30/1 -> adder1/2(In2)
  Selector3/1 -> delayMatch5/1
  Selector/1 -> delayMatch10/1
  Selector1/1 -> delayMatch13/1
  delayMatch16/1 -> multiplier8/2(In2)
  delayMatch25/1 -> multiplier11/2(In2)
  delayMatch17/1 -> multiplier9/2(In2)
  delayMatch23/1 -> multiplier10/2(In2)
  delayMatch/1 -> delayMatch18/1
  delayMatch1/1 -> delayMatch19/1
  delayMatch2/1 -> delayMatch21/1
  delayMatch3/1 -> delayMatch22/1
  delayMatch31/1 -> multiplier6/2(In2)
  delayMatch5/1 -> delayMatch24/1
  delayMatch4/1 -> delayMatch26/1
  delayMatch6/1 -> delayMatch27/1
  delayMatch7/1 -> delayMatch28/1
  delayMatch8/1 -> delayMatch29/1
  delayMatch9/1 -> delayMatch30/1
  delayMatch35/1 -> multiplier7/2(In2)
  delayMatch10/1 -> delayMatch32/1
  delayMatch11/1 -> delayMatch33/1
  delayMatch12/1 -> delayMatch34/1
  delayMatch13/1 -> delayMatch36/1
  delayMatch14/1 -> delayMatch37/1
  delayMatch15/1 -> delayMatch38/1
  SampleTime_div_Ld/1 -> delayMatch2/1
  SampleTime_div_Lq/1 -> delayMatch8/1
  SampleTime_div_Lx/1 -> delayMatch11/1
  SampleTime_div_Ly/1 -> delayMatch14/1
  last_applied_optimal_voltage_vector/1 -> Reshape/1
  id_measured/1 -> delayMatch3/1, multiplier11/1(In1), multiplier9/1(In1)
  iq_measured/1 -> delayMatch9/1, delayMatch1/1, multiplier10/1(In1)
  ix_measured/1 -> delayMatch12/1, multiplier6/1(In1)
  iy_measured/1 -> delayMatch15/1, multiplier7/1(In1)
  psiPM/1 -> delayMatch4/1
  Lq/1 -> delayMatch16/1
  Ld/1 -> delayMatch25/1
  Rs/1 -> delayMatch35/1, delayMatch31/1, delayMatch23/1, delayMatch17/1
  omega_el/1 -> delayMatch6/1, multiplier8/1(In1)

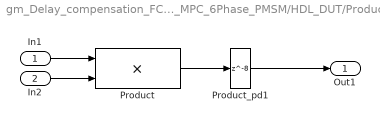
== system gm_Delay_compensation_FCS_MPC_6Phase_PMSM/HDL_DUT/Product ==
  In1 : Inport
  In2 : Inport  Port=2
  Product : Product  Inputs=**  OutDataTypeStr=single  SampleTime=1e-08
  Product_pd1 : Delay  DelayLength=8
  Out1 : Outport
  wires:
  In1/1 -> Product/1
  In2/1 -> Product/2
  Product/1 -> Product_pd1/1
  Product_pd1/1 -> Out1/1

== system gm_Delay_compensation_FCS_MPC_6Phase_PMSM/HDL_DUT/Detect Rise Positive/Positive ==
  u : Inport  OutDataTypeStr=boolean  SampleTime=1e-08
  Compare : RelationalOperator  Operator=>  OutDataTypeStr=boolean  ZeroCross=off
  Constant : Constant  DisableCoverage=on  Value=0  OutDataTypeStr=Inherit: Inherit via back propagation  SampleTime=-1  PreserveConstantTs=on
  y : Outport  SampleTime=1e-08
  wires:
  Compare/1 -> y/1
  Constant/1 -> Compare/2
  u/1 -> Compare/1

== system gm_Delay_compensation_FCS_MPC_6Phase_PMSM/HDL_DUT/Detect Rise Positive1/Positive ==
  u : Inport  OutDataTypeStr=boolean  SampleTime=1e-08
  Compare : RelationalOperator  Operator=>  OutDataTypeStr=boolean  ZeroCross=off
  Constant : Constant  DisableCoverage=on  Value=0  OutDataTypeStr=Inherit: Inherit via back propagation  SampleTime=-1  PreserveConstantTs=on
  y : Outport  SampleTime=1e-08
  wires:
  Compare/1 -> y/1
  Constant/1 -> Compare/2
  u/1 -> Compare/1

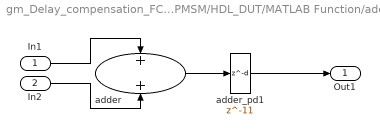
== system gm_Delay_compensation_FCS_MPC_6Phase_PMSM/HDL_DUT/MATLAB Function/adder ==
  In1 : Inport
  In2 : Inport  Port=2
  adder : Sum  OutDataTypeStr=single  SampleTime=1e-08
  adder_pd1 : Delay  DelayLength=11
  Out1 : Outport
  wires:
  In1/1 -> adder/1
  In2/1 -> adder/2
  adder/1 -> adder_pd1/1
  adder_pd1/1 -> Out1/1

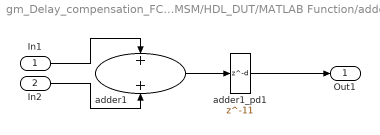
== system gm_Delay_compensation_FCS_MPC_6Phase_PMSM/HDL_DUT/MATLAB Function/adder1 ==
  In1 : Inport
  In2 : Inport  Port=2
  adder1 : Sum  OutDataTypeStr=single  SampleTime=1e-08
  adder1_pd1 : Delay  DelayLength=11
  Out1 : Outport
  wires:
  In1/1 -> adder1/1
  In2/1 -> adder1/2
  adder1/1 -> adder1_pd1/1
  adder1_pd1/1 -> Out1/1

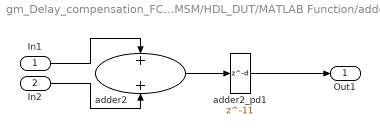
== system gm_Delay_compensation_FCS_MPC_6Phase_PMSM/HDL_DUT/MATLAB Function/adder2 ==
  In1 : Inport
  In2 : Inport  Port=2
  adder2 : Sum  OutDataTypeStr=single  SampleTime=1e-08
  adder2_pd1 : Delay  DelayLength=11
  Out1 : Outport
  wires:
  In1/1 -> adder2/1
  In2/1 -> adder2/2
  adder2/1 -> adder2_pd1/1
  adder2_pd1/1 -> Out1/1

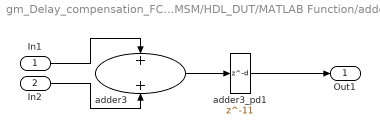
== system gm_Delay_compensation_FCS_MPC_6Phase_PMSM/HDL_DUT/MATLAB Function/adder3 ==
  In1 : Inport
  In2 : Inport  Port=2
  adder3 : Sum  OutDataTypeStr=single  SampleTime=1e-08
  adder3_pd1 : Delay  DelayLength=11
  Out1 : Outport
  wires:
  In1/1 -> adder3/1
  In2/1 -> adder3/2
  adder3/1 -> adder3_pd1/1
  adder3_pd1/1 -> Out1/1

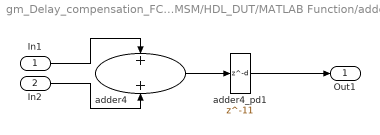
== system gm_Delay_compensation_FCS_MPC_6Phase_PMSM/HDL_DUT/MATLAB Function/adder4 ==
  In1 : Inport
  In2 : Inport  Port=2
  adder4 : Sum  OutDataTypeStr=single  SampleTime=1e-08
  adder4_pd1 : Delay  DelayLength=11
  Out1 : Outport
  wires:
  In1/1 -> adder4/1
  In2/1 -> adder4/2
  adder4/1 -> adder4_pd1/1
  adder4_pd1/1 -> Out1/1

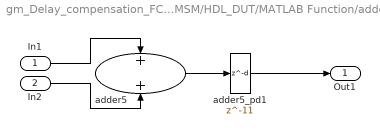
== system gm_Delay_compensation_FCS_MPC_6Phase_PMSM/HDL_DUT/MATLAB Function/adder5 ==
  In1 : Inport
  In2 : Inport  Port=2
  adder5 : Sum  OutDataTypeStr=single  SampleTime=1e-08
  adder5_pd1 : Delay  DelayLength=11
  Out1 : Outport
  wires:
  In1/1 -> adder5/1
  In2/1 -> adder5/2
  adder5/1 -> adder5_pd1/1
  adder5_pd1/1 -> Out1/1

== system gm_Delay_compensation_FCS_MPC_6Phase_PMSM/HDL_DUT/MATLAB Function/multiplier ==
  In1 : Inport
  In2 : Inport  Port=2
  multiplier : Product  Inputs=**  OutDataTypeStr=single  SampleTime=1e-08
  multiplier_pd1 : Delay  DelayLength=8
  Out1 : Outport
  wires:
  In1/1 -> multiplier/1
  In2/1 -> multiplier/2
  multiplier/1 -> multiplier_pd1/1
  multiplier_pd1/1 -> Out1/1

== system gm_Delay_compensation_FCS_MPC_6Phase_PMSM/HDL_DUT/MATLAB Function/multiplier1 ==
  In1 : Inport
  In2 : Inport  Port=2
  multiplier1 : Product  Inputs=**  OutDataTypeStr=single  SampleTime=1e-08
  multiplier1_pd1 : Delay  DelayLength=8
  Out1 : Outport
  wires:
  In1/1 -> multiplier1/1
  In2/1 -> multiplier1/2
  multiplier1/1 -> multiplier1_pd1/1
  multiplier1_pd1/1 -> Out1/1

== system gm_Delay_compensation_FCS_MPC_6Phase_PMSM/HDL_DUT/MATLAB Function/multiplier10 ==
  In1 : Inport
  In2 : Inport  Port=2
  multiplier10 : Product  Inputs=**  OutDataTypeStr=single  SampleTime=1e-08
  multiplier10_pd1 : Delay  DelayLength=8
  Out1 : Outport
  wires:
  In1/1 -> multiplier10/1
  In2/1 -> multiplier10/2
  multiplier10/1 -> multiplier10_pd1/1
  multiplier10_pd1/1 -> Out1/1

== system gm_Delay_compensation_FCS_MPC_6Phase_PMSM/HDL_DUT/MATLAB Function/multiplier11 ==
  In1 : Inport
  In2 : Inport  Port=2
  multiplier11 : Product  Inputs=**  OutDataTypeStr=single  SampleTime=1e-08
  multiplier11_pd1 : Delay  DelayLength=8
  Out1 : Outport
  wires:
  In1/1 -> multiplier11/1
  In2/1 -> multiplier11/2
  multiplier11/1 -> multiplier11_pd1/1
  multiplier11_pd1/1 -> Out1/1

== system gm_Delay_compensation_FCS_MPC_6Phase_PMSM/HDL_DUT/MATLAB Function/multiplier2 ==
  In1 : Inport
  In2 : Inport  Port=2
  multiplier2 : Product  Inputs=**  OutDataTypeStr=single  SampleTime=1e-08
  multiplier2_pd1 : Delay  DelayLength=8
  Out1 : Outport
  wires:
  In1/1 -> multiplier2/1
  In2/1 -> multiplier2/2
  multiplier2/1 -> multiplier2_pd1/1
  multiplier2_pd1/1 -> Out1/1

== system gm_Delay_compensation_FCS_MPC_6Phase_PMSM/HDL_DUT/MATLAB Function/multiplier3 ==
  In1 : Inport
  In2 : Inport  Port=2
  multiplier3 : Product  Inputs=**  OutDataTypeStr=single  SampleTime=1e-08
  multiplier3_pd1 : Delay  DelayLength=8
  Out1 : Outport
  wires:
  In1/1 -> multiplier3/1
  In2/1 -> multiplier3/2
  multiplier3/1 -> multiplier3_pd1/1
  multiplier3_pd1/1 -> Out1/1

== system gm_Delay_compensation_FCS_MPC_6Phase_PMSM/HDL_DUT/MATLAB Function/multiplier4 ==
  In1 : Inport
  In2 : Inport  Port=2
  multiplier4 : Product  Inputs=**  OutDataTypeStr=single  SampleTime=1e-08
  multiplier4_pd1 : Delay  DelayLength=8
  Out1 : Outport
  wires:
  In1/1 -> multiplier4/1
  In2/1 -> multiplier4/2
  multiplier4/1 -> multiplier4_pd1/1
  multiplier4_pd1/1 -> Out1/1

== system gm_Delay_compensation_FCS_MPC_6Phase_PMSM/HDL_DUT/MATLAB Function/multiplier5 ==
  In1 : Inport
  In2 : Inport  Port=2
  multiplier5 : Product  Inputs=**  OutDataTypeStr=single  SampleTime=1e-08
  multiplier5_pd1 : Delay  DelayLength=8
  Out1 : Outport
  wires:
  In1/1 -> multiplier5/1
  In2/1 -> multiplier5/2
  multiplier5/1 -> multiplier5_pd1/1
  multiplier5_pd1/1 -> Out1/1

== system gm_Delay_compensation_FCS_MPC_6Phase_PMSM/HDL_DUT/MATLAB Function/multiplier6 ==
  In1 : Inport
  In2 : Inport  Port=2
  multiplier6 : Product  Inputs=**  OutDataTypeStr=single  SampleTime=1e-08
  multiplier6_pd1 : Delay  DelayLength=8
  Out1 : Outport
  wires:
  In1/1 -> multiplier6/1
  In2/1 -> multiplier6/2
  multiplier6/1 -> multiplier6_pd1/1
  multiplier6_pd1/1 -> Out1/1

== system gm_Delay_compensation_FCS_MPC_6Phase_PMSM/HDL_DUT/MATLAB Function/multiplier7 ==
  In1 : Inport
  In2 : Inport  Port=2
  multiplier7 : Product  Inputs=**  OutDataTypeStr=single  SampleTime=1e-08
  multiplier7_pd1 : Delay  DelayLength=8
  Out1 : Outport
  wires:
  In1/1 -> multiplier7/1
  In2/1 -> multiplier7/2
  multiplier7/1 -> multiplier7_pd1/1
  multiplier7_pd1/1 -> Out1/1

== system gm_Delay_compensation_FCS_MPC_6Phase_PMSM/HDL_DUT/MATLAB Function/multiplier8 ==
  In1 : Inport
  In2 : Inport  Port=2
  multiplier8 : Product  Inputs=**  OutDataTypeStr=single  SampleTime=1e-08
  multiplier8_pd1 : Delay  DelayLength=8
  Out1 : Outport
  wires:
  In1/1 -> multiplier8/1
  In2/1 -> multiplier8/2
  multiplier8/1 -> multiplier8_pd1/1
  multiplier8_pd1/1 -> Out1/1

== system gm_Delay_compensation_FCS_MPC_6Phase_PMSM/HDL_DUT/MATLAB Function/multiplier9 ==
  In1 : Inport
  In2 : Inport  Port=2
  multiplier9 : Product  Inputs=**  OutDataTypeStr=single  SampleTime=1e-08
  multiplier9_pd1 : Delay  DelayLength=8
  Out1 : Outport
  wires:
  In1/1 -> multiplier9/1
  In2/1 -> multiplier9/2
  multiplier9/1 -> multiplier9_pd1/1
  multiplier9_pd1/1 -> Out1/1

== system gm_Delay_compensation_FCS_MPC_6Phase_PMSM/HDL_DUT/MATLAB Function/subtract ==
  In1 : Inport
  In2 : Inport  Port=2
  subtract : Sum  Inputs=+-  OutDataTypeStr=single  SampleTime=1e-08
  subtract_pd1 : Delay  DelayLength=11
  Out1 : Outport
  wires:
  In1/1 -> subtract/1
  In2/1 -> subtract/2
  subtract/1 -> subtract_pd1/1
  subtract_pd1/1 -> Out1/1

== system gm_Delay_compensation_FCS_MPC_6Phase_PMSM/HDL_DUT/MATLAB Function/subtract1 ==
  In1 : Inport
  In2 : Inport  Port=2
  subtract1 : Sum  Inputs=+-  OutDataTypeStr=single  SampleTime=1e-08
  subtract1_pd1 : Delay  DelayLength=11
  Out1 : Outport
  wires:
  In1/1 -> subtract1/1
  In2/1 -> subtract1/2
  subtract1/1 -> subtract1_pd1/1
  subtract1_pd1/1 -> Out1/1

== system gm_Delay_compensation_FCS_MPC_6Phase_PMSM/HDL_DUT/MATLAB Function/subtract2 ==
  In1 : Inport
  In2 : Inport  Port=2
  subtract2 : Sum  Inputs=+-  OutDataTypeStr=single  SampleTime=1e-08
  subtract2_pd1 : Delay  DelayLength=11
  Out1 : Outport
  wires:
  In1/1 -> subtract2/1
  In2/1 -> subtract2/2
  subtract2/1 -> subtract2_pd1/1
  subtract2_pd1/1 -> Out1/1

== system gm_Delay_compensation_FCS_MPC_6Phase_PMSM/HDL_DUT/MATLAB Function/subtract3 ==
  In1 : Inport
  In2 : Inport  Port=2
  subtract3 : Sum  Inputs=+-  OutDataTypeStr=single  SampleTime=1e-08
  subtract3_pd1 : Delay  DelayLength=11
  Out1 : Outport
  wires:
  In1/1 -> subtract3/1
  In2/1 -> subtract3/2
  subtract3/1 -> subtract3_pd1/1
  subtract3_pd1/1 -> Out1/1

== system gm_Delay_compensation_FCS_MPC_6Phase_PMSM/HDL_DUT/MATLAB Function/subtract4 ==
  In1 : Inport
  In2 : Inport  Port=2
  subtract4 : Sum  Inputs=+-  OutDataTypeStr=single  SampleTime=1e-08
  subtract4_pd1 : Delay  DelayLength=11
  Out1 : Outport
  wires:
  In1/1 -> subtract4/1
  In2/1 -> subtract4/2
  subtract4/1 -> subtract4_pd1/1
  subtract4_pd1/1 -> Out1/1
